simulink model "Simulation"  (R2020b)
settings: Solver=VariableStepAuto  StartTime=0.0  StopTime=10  RelTol=1e-3
libraries: vrlib x1
settings Model: Creator=vorps  LastModifiedBy=vorps

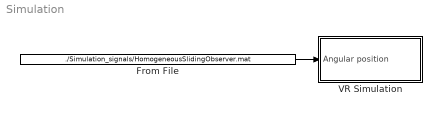
== system Simulation ==
  From File : FromFile  FileName=./Simulation_signals/HomogeneousSlidingObserver.mat  SampleTime=0.001
  VR Simulation : Subsystem
  wires:
  From File/1 -> VR Simulation/1(Angular position)

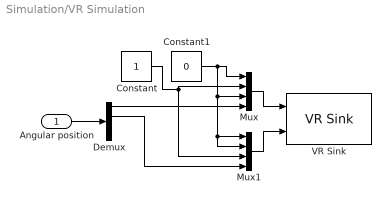
== system Simulation/VR Simulation ==
  Angular position : Inport
  Constant : Constant
  Constant1 : Constant  Value=0
  Demux : Demux
  Mux : Mux
  Mux1 : Mux
  VR Sink : vrlib/VR Sink  InstantiateOnLoad=on  SampleTime=0.01  ViewEnable=on  RemoteChange=off  RemoteView=off  FieldsWritten=Rotary_Arm.rotation.4.1.1.double#Pendulum.rotation.4.1.1.double  WorldFileName=/home/vorps/Documents/Etude/M2/Projet/Modelling/Pendulum.x3d  AutoView=off  VideoDimensions=[]  AllowVariableSize=off
  wires:
  Constant1/1 -> Mux1/2, Mux1/1, Mux/3, Mux/1
  Demux/1 -> Mux/4
  Mux1/1 -> VR Sink/2
  Mux/1 -> VR Sink/1
  Constant/1 -> Mux1/3, Mux/2
  Angular position/1 -> Demux/1
  Demux/2 -> Mux1/4
